simulink model "NPSS_Sfunction"  (Simulink 7.5)
settings: Solver=FixedStepDiscrete  StartTime=0.0  StopTime=10  FixedStep=0.02  RelTol=1e-3
InitFcn:
  | setup_NPSS_Simulink
undefined symbols (not defined in the file or in its folder): in
libraries: simulink x1
settings Model: Creator=jcsank  LastModifiedBy=jcchin

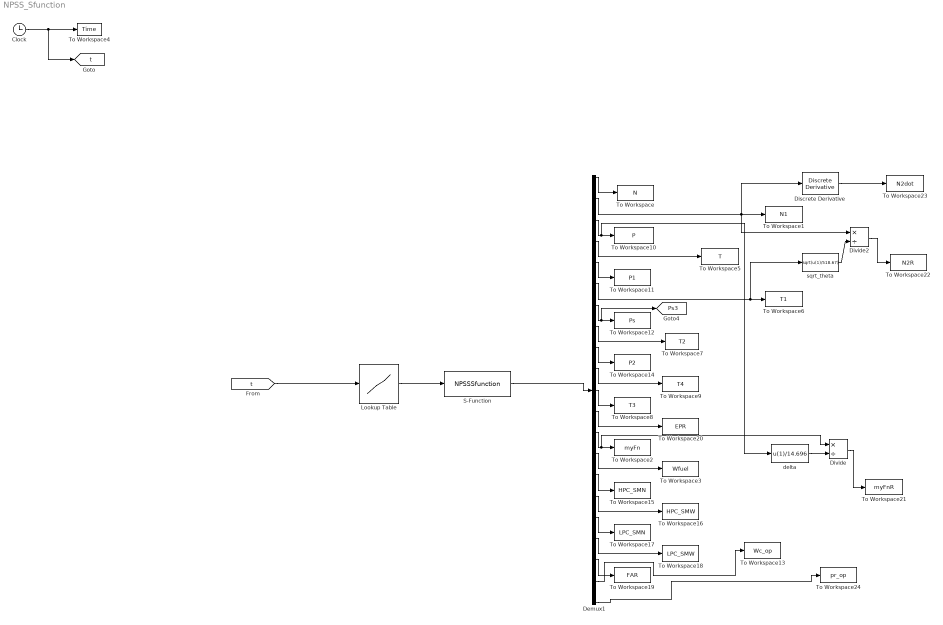
== system NPSS_Sfunction ==
  Clock : Clock
      settings: Decimation=10
  Demux1 : Demux  Outputs=21
  Discrete Derivative : simulink/Discrete/Discrete Derivative  SystemSampleTime=-1  gainval=1.0  ICPrevScaledInput=0.0  OutMin=[]  OutMax=[]  OutDataType=fixdt(1, 16)  OutScaling=2^-10  DoSatur=off
  Divide : Product  Inputs=*/
  Divide2 : Product  Inputs=*/
  Lookup Table : Lookup  InputValues=in.t  Table=in.wf
  S-Function : S-Function  FunctionName=NPSSSfunction  Parameters='150_PAX_Sfunction.config'  EnableBusSupport=off
  To Workspace : ToWorkspace  VariableName=N  SampleTime=-1  SaveFormat=Array
  To Workspace1 : ToWorkspace  VariableName=N1  SampleTime=-1  SaveFormat=Array
  To Workspace10 : ToWorkspace  VariableName=P  SampleTime=-1  SaveFormat=Array
  To Workspace11 : ToWorkspace  VariableName=P1  SampleTime=-1  SaveFormat=Array
  To Workspace12 : ToWorkspace  VariableName=Ps  SampleTime=-1  SaveFormat=Array
  To Workspace13 : ToWorkspace  VariableName=Wc_op  SampleTime=-1  SaveFormat=Array
  To Workspace14 : ToWorkspace  VariableName=P2  SampleTime=-1  SaveFormat=Array
  To Workspace15 : ToWorkspace  VariableName=HPC_SMN  SampleTime=-1  SaveFormat=Array
  To Workspace16 : ToWorkspace  VariableName=HPC_SMW  SampleTime=-1  SaveFormat=Array
  To Workspace17 : ToWorkspace  VariableName=LPC_SMN  SampleTime=-1  SaveFormat=Array
  To Workspace18 : ToWorkspace  VariableName=LPC_SMW  SampleTime=-1  SaveFormat=Array
  To Workspace19 : ToWorkspace  VariableName=FAR  SampleTime=-1  SaveFormat=Array
  To Workspace2 : ToWorkspace  VariableName=myFn  SampleTime=-1  SaveFormat=Array
  To Workspace20 : ToWorkspace  VariableName=EPR  SampleTime=-1  SaveFormat=Array
  To Workspace21 : ToWorkspace  VariableName=myFnR  SampleTime=-1  SaveFormat=Array
  To Workspace22 : ToWorkspace  VariableName=N2R  SampleTime=-1  SaveFormat=Array
  To Workspace23 : ToWorkspace  VariableName=N2dot  SampleTime=-1  SaveFormat=Array
  To Workspace24 : ToWorkspace  VariableName=pr_op  SampleTime=-1  SaveFormat=Array
  To Workspace3 : ToWorkspace  VariableName=Wfuel  SampleTime=-1  SaveFormat=Array
  To Workspace4 : ToWorkspace  VariableName=Time  SampleTime=-1  SaveFormat=Array
  To Workspace5 : ToWorkspace  VariableName=T  SampleTime=-1  SaveFormat=Array
  To Workspace6 : ToWorkspace  VariableName=T1  SampleTime=-1  SaveFormat=Array
  To Workspace7 : ToWorkspace  VariableName=T2  SampleTime=-1  SaveFormat=Array
  To Workspace8 : ToWorkspace  VariableName=T3  SampleTime=-1  SaveFormat=Array
  To Workspace9 : ToWorkspace  VariableName=T4  SampleTime=-1  SaveFormat=Array
  delta : Fcn  Expr=u(1)/14.696
  sqrt_theta : Fcn  Expr=sqrt(u(1)/518.67)
  tag scope: Ps3=global, t=global
  wires:
  Lookup Table/1 -> S-Function/1
  Clock/1 -> [t], To Workspace4/1
  [t] -> Lookup Table/1
  Divide/1 -> To Workspace21/1
  delta/1 -> Divide/2
  Divide2/1 -> To Workspace22/1
  Discrete Derivative/1 -> To Workspace23/1
  Demux1/1 -> To Workspace/1
  Demux1/2 -> To Workspace1/1, Discrete Derivative/1, Divide2/1
  Demux1/3 -> To Workspace10/1, delta/1
  Demux1/4 -> To Workspace5/1
  Demux1/5 -> To Workspace11/1
  Demux1/6 -> To Workspace6/1, sqrt_theta/1
  Demux1/7 -> To Workspace12/1, [Ps3]
  Demux1/8 -> To Workspace7/1
  Demux1/10 -> To Workspace9/1
  Demux1/9 -> To Workspace14/1
  Demux1/11 -> To Workspace8/1
  Demux1/12 -> To Workspace20/1
  Demux1/13 -> To Workspace2/1, Divide/1
  Demux1/14 -> To Workspace3/1
  Demux1/15 -> To Workspace15/1
  Demux1/16 -> To Workspace16/1
  Demux1/17 -> To Workspace17/1
  Demux1/18 -> To Workspace18/1
  Demux1/19 -> To Workspace19/1
  sqrt_theta/1 -> Divide2/2
  S-Function/1 -> Demux1/1
  Demux1/20 -> To Workspace13/1
  Demux1/21 -> To Workspace24/1
